simulink model "W_server_mock_oClientServer_Model"  (R2024b)
settings: Solver=FixedStepDiscrete  StartTime=0.0  StopTime=10.0  FixedStep=0.05  RelTol=1e-3
settings Model: Tag=EP_AA_WRAPPER_SERVER_FUNCTIONS_MOCK  DataDictionary=Wrapper_oClientServer_Model.sldd  Creator=nabilekhoury  LastModifiedBy=nabilekhoury
settings OptimizationCC: DefaultParameterBehavior=Inlined  OptimizeBlockIOStorage=off  BufferReuse=off  ReuseModelBlockBuffer=off  GlobalBufferReuse=off  ExpressionFolding=off  EnableMemcpy=off  PassReuseOutputArgsAs=Individual arguments  LocalBlockOutputs=off  ZeroExternalMemoryAtStartup=off  ZeroInternalMemoryAtStartup=off  OptimizeDataStoreBuffers=off  BusAssignmentInplaceUpdate=off  OptimizationLevel=level0  OptimizationCustomize=off  EfficientTunableParamExpr=on
settings DebuggingCC: ParameterTunabilityLossMsg=error
settings ModelReferenceCC: ModelReferenceNumInstancesAllowed=Single
settings SFSimCC: MATLABDynamicMemAlloc=off  SimTargetLang=C++
settings RTWCC: Description=Embedded Coder  SystemTargetFile=ert.tlc  GenCodeOnly=on  TemplateMakefile=ert_default_tmf  TargetLang=C++
settings CodeAppCC: ForceParamTrailComments=on  IgnoreCustomStorageClasses=off  MaxIdLength=256  OperatorAnnotations=on  SimulinkDataObjDesc=on  SFDataObjDesc=on  CustomSymbolStrGlobalVar=w_$R$N$M  CustomSymbolStrType=w_$N$R$M_T  InsertBlockDesc=on
settings ERTTargetCC: TargetLangStandard=C++17 (ISO)  GenerateSampleERTMain=on  SupportAbsoluteTime=off  SupportNonFinite=off  SupportComplex=off  RootIOFormat=Structure reference  ERTCustomFileTemplate=example_file_process.tlc

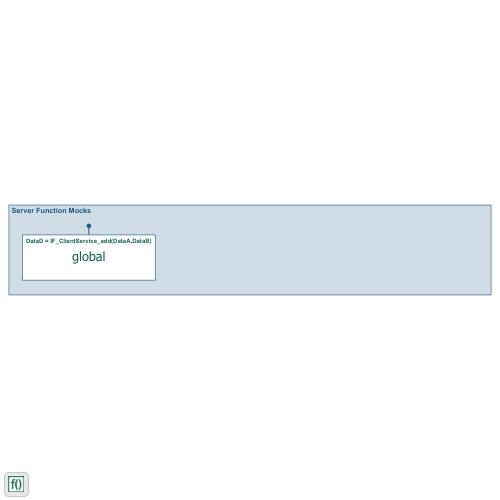
[thumbnail: Simulink's stored preview of the top-level diagram]
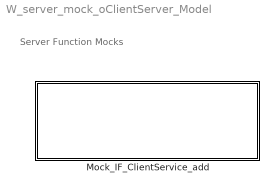
== system W_server_mock_oClientServer_Model ==
  note: Server Function Mocks
  Mock_IF_ClientService_add : Subsystem  TreatAsAtomicUnit=on

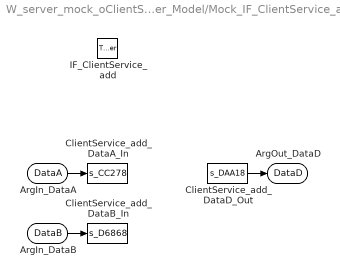
== system W_server_mock_oClientServer_Model/Mock_IF_ClientService_add ==
  IF_ClientService_add : TriggerPort  TriggerType=function-call  IsSimulinkFunction=on  FunctionName=IF_ClientService_add  ScopeName=ClientService  VariantControl=(inherit)
  ClientService_add_DataA_In : DataStoreWrite  DataStoreName=s_CC278  IndexOptions=Index vector (dialog)  Indices=1  OutputSizes=1
  ClientService_add_DataB_In : DataStoreWrite  DataStoreName=s_D6868  IndexOptions=Index vector (dialog)  Indices=1  OutputSizes=1
  ClientService_add_DataD_Out : DataStoreRead  DataStoreName=s_DAA18  IndexOptions=Index vector (dialog)  Indices=1  OutputSizes=1
  ArgIn_DataA : ArgIn  PortDimensions=[1 1]  ArgumentName=DataA
  ArgIn_DataB : ArgIn  Port=2  PortDimensions=[1 1]  ArgumentName=DataB
  ArgOut_DataD : ArgOut  PortDimensions=[1 1]  ArgumentName=DataD
  wires:
  ArgIn_DataA/1 -> ClientService_add_DataA_In/1
  ArgIn_DataB/1 -> ClientService_add_DataB_In/1
  ClientService_add_DataD_Out/1 -> ArgOut_DataD/1
